simulink model "GisooLib"  (Simulink 8.1)
settings: Solver=ode45  StartTime=0.0  StopTime=10.0  RelTol=1e-3
libraries: commutil2 x54, xpclib x9, simulink x7, etargetslib x7, dspnetwork x7, GisooLib x1, commcrc2 x1
settings Model: Creator=behdad  LastModifiedBy=behdad
settings DataIOCC: SignalLoggingSaveFormat=Dataset
settings OptimizationCC: ExpressionDepthLimit=128
settings DebuggingCC: FcnCallInpInsideContextMsg=EnableAllAsError
settings GRTTargetCC: CombineOutputUpdateFcns=on  GRTInterface=off

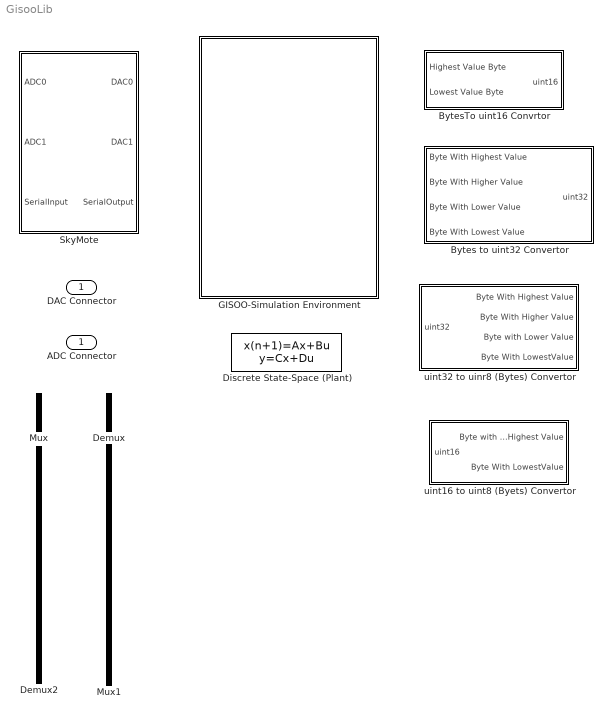
== system GisooLib ==
  ADC Connector : Inport
  Bytes to uint32 Convertor : Subsystem
  BytesTo uint16 Convrtor : Subsystem
  Demux : Demux  Outputs=2
  Demux2 : Demux  Outputs=16
  Discrete State-Space (Plant) : DiscreteStateSpace
  GISOO-Simulation Environment : Subsystem  TreatAsAtomicUnit=on
  Mux : Mux  Inputs=2
  Mux1 : Mux  Inputs=16
  SkyMote : Subsystem  mask{moteID=1, PacketType=6}
      mask prompts: PacketType "Serial Packet Type (Required block receives Serial data):"
  uint16 to uint8 (Byets) Convertor : Subsystem
  uint32 to uinr8 (Bytes) Convertor : Subsystem
  DAC Connector : Outport

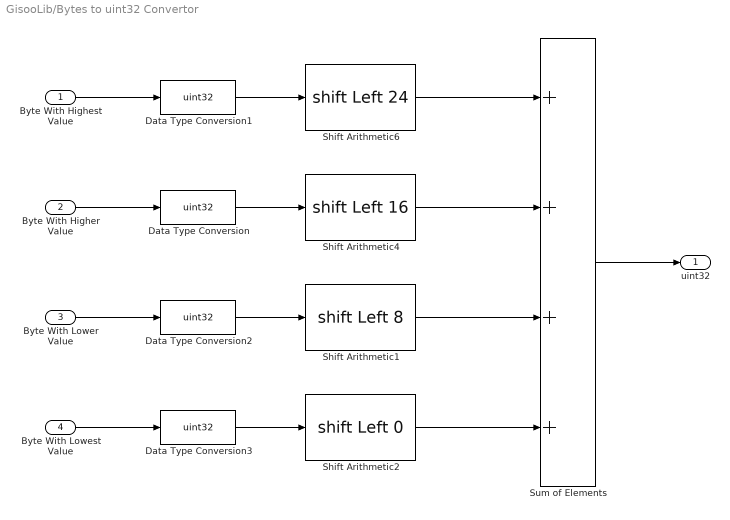
== system GisooLib/Bytes to uint32 Convertor ==
  Byte With Highest Value : Inport
  Byte With Higher Value : Inport  Port=2
  Byte With Lower Value : Inport  Port=3
  Byte With Lowest Value : Inport  Port=4
  Data Type Conversion{,1..3} (4 alike) : DataTypeConversion  OutDataTypeStr=uint32
  Shift Arithmetic1 : ArithShift  BitShiftNumber=8  BitShiftDirection=Left
  Shift Arithmetic2 : ArithShift  BitShiftDirection=Left
  Shift Arithmetic4 : ArithShift  BitShiftNumber=16  BitShiftDirection=Left
  Shift Arithmetic6 : ArithShift  BitShiftNumber=24  BitShiftDirection=Left
  Sum of Elements : Sum  Inputs=++++  CollapseDim=4  AccumDataTypeStr=uint8  OutDataTypeStr=uint32  InputSameDT=on
  uint32 : Outport
  wires:
  Data Type Conversion3/1 -> Shift Arithmetic2/1
  Shift Arithmetic1/1 -> Sum of Elements/3
  Shift Arithmetic6/1 -> Sum of Elements/1
  Byte With Lowest Value/1 -> Data Type Conversion3/1
  Shift Arithmetic2/1 -> Sum of Elements/4
  Byte With Lower Value/1 -> Data Type Conversion2/1
  Data Type Conversion2/1 -> Shift Arithmetic1/1
  Shift Arithmetic4/1 -> Sum of Elements/2
  Byte With Higher Value/1 -> Data Type Conversion/1
  Byte With Highest Value/1 -> Data Type Conversion1/1
  Data Type Conversion/1 -> Shift Arithmetic4/1
  Data Type Conversion1/1 -> Shift Arithmetic6/1
  Sum of Elements/1 -> uint32/1

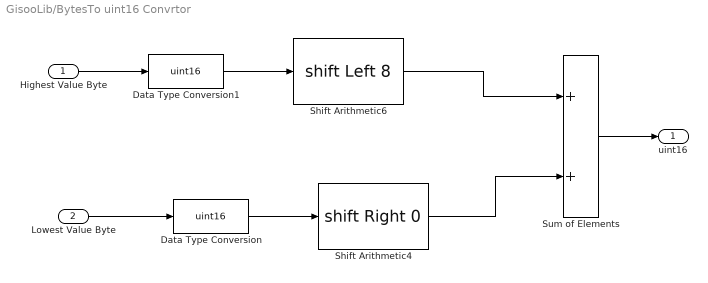
== system GisooLib/BytesTo uint16 Convrtor ==
  Highest Value Byte : Inport
  Lowest Value Byte : Inport  Port=2
  Data Type Conversion : DataTypeConversion  OutDataTypeStr=uint16
  Data Type Conversion1 : DataTypeConversion  OutDataTypeStr=uint16
  Shift Arithmetic4 : ArithShift  BitShiftDirection=Right
  Shift Arithmetic6 : ArithShift  BitShiftNumber=8  BitShiftDirection=Left
  Sum of Elements : Sum  CollapseDim=4  OutDataTypeStr=uint16
  uint16 : Outport
  wires:
  Lowest Value Byte/1 -> Data Type Conversion/1
  Highest Value Byte/1 -> Data Type Conversion1/1
  Data Type Conversion/1 -> Shift Arithmetic4/1
  Data Type Conversion1/1 -> Shift Arithmetic6/1
  Sum of Elements/1 -> uint16/1
  Shift Arithmetic4/1 -> Sum of Elements/2
  Shift Arithmetic6/1 -> Sum of Elements/1

== system GisooLib/GISOO-Simulation Environment ==
  CoojaConnector : Subsystem
  SynchronizerLoop : WhileIterator  MaxIters=-1  WhileBlockType=do-while  ShowIterationPort=on
  wires:
  CoojaConnector/1(Wait) -> SynchronizerLoop/1
  SynchronizerLoop/1 -> CoojaConnector/1(DelayNum.)

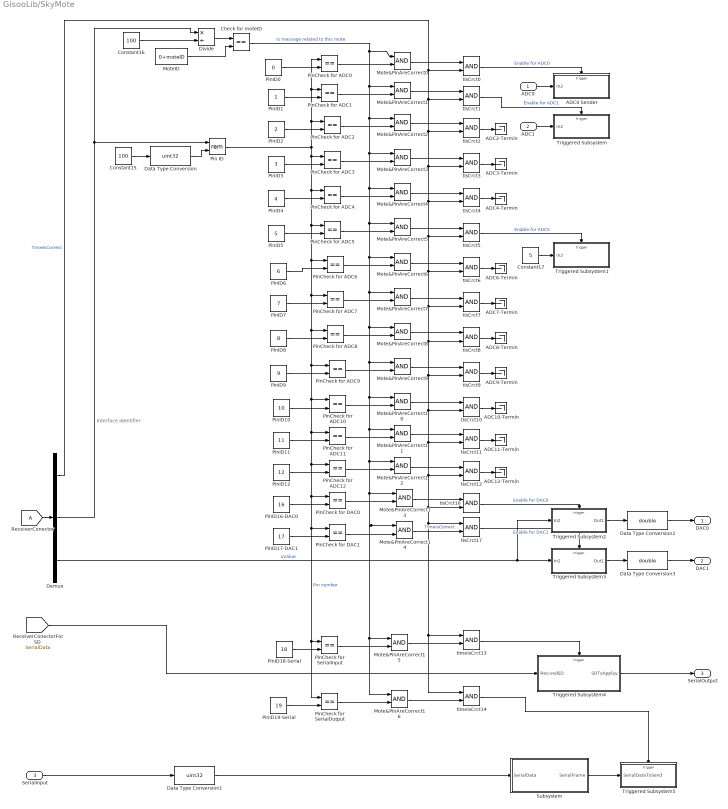
== system GisooLib/SkyMote ==
  note: Interface Identifier
  ADC0 : Inport
  ADC1 : Inport  Port=2
  SerialInput : Inport  Port=3
  ADC0 Sender : Subsystem  TreatAsAtomicUnit=on
  ADC10-Termin : Terminator
  ADC11-Termin : Terminator
  ADC12-Termin : Terminator
  ADC2-Termin : Terminator
  ADC3-Termin : Terminator
  ADC4-Termin : Terminator
  ADC6-Termin : Terminator
  ADC7-Termin : Terminator
  ADC8-Termin : Terminator
  ADC9-Termin : Terminator
  Check for moteID : RelationalOperator  Operator===  OutDataTypeStr=boolean
  Constant15 : Constant  Value=100
  Constant16 : Constant  Value=100
  Constant17 : Constant  Value=5
  Data Type Conversion : DataTypeConversion  OutDataTypeStr=uint32
  Data Type Conversion1 : DataTypeConversion  OutDataTypeStr=uint32
  Data Type Conversion2 : DataTypeConversion  OutDataTypeStr=double
  Data Type Conversion3 : DataTypeConversion  OutDataTypeStr=double
  Demux : Demux  Outputs=3
  Divide : Product  Inputs=*/  OutDataTypeStr=int32
  Mote&PinAreCorrect{0..16} (17 alike) : Logic  AllPortsSameDT=off  OutDataTypeStr=boolean
  MoteID : Constant  Value=0+moteID
  Pin ID : Math  Operator=rem  SaturateOnIntegerOverflow=on
  PinCheck for ADC{0..12} (13 alike) : RelationalOperator  Operator===  OutDataTypeStr=boolean
  PinCheck for DAC0 : RelationalOperator  Operator===  OutDataTypeStr=boolean
  PinCheck for DAC1 : RelationalOperator  Operator===  OutDataTypeStr=boolean
  PinCheck for SerialInput : RelationalOperator  Operator===  OutDataTypeStr=boolean
  PinCheck for SerialOutput : RelationalOperator  Operator===  OutDataTypeStr=boolean
  PinID0 : Constant  Value=0
  PinID1 : Constant
  PinID10 : Constant  Value=10
  PinID11 : Constant  Value=11
  PinID12 : Constant  Value=12
  PinID16-DAC0 : Constant  Value=16
  PinID17-DAC1 : Constant  Value=17
  PinID18-Serial : Constant  Value=18
  PinID19-Serial : Constant  Value=19
  PinID2 : Constant  Value=2
  PinID3 : Constant  Value=3
  PinID4 : Constant  Value=4
  PinID5 : Constant  Value=5
  PinID6 : Constant  Value=6
  PinID7 : Constant  Value=7
  PinID8 : Constant  Value=8
  PinID9 : Constant  Value=9
  Subsystem : Subsystem
  Triggered Subsystem : Subsystem  TreatAsAtomicUnit=on
  Triggered Subsystem1 : Subsystem  TreatAsAtomicUnit=on
  Triggered Subsystem2 : Subsystem  TreatAsAtomicUnit=on
  Triggered Subsystem3 : Subsystem  TreatAsAtomicUnit=on
  Triggered Subsystem4 : Subsystem  TreatAsAtomicUnit=on
  Triggered Subsystem5 : Subsystem  TreatAsAtomicUnit=on
  tIsCrct{0..12,16..17} (15 alike) : Logic  AllPortsSameDT=off  OutDataTypeStr=boolean
  timeIsCrct13 : Logic  AllPortsSameDT=off  OutDataTypeStr=boolean
  timeIsCrct14 : Logic  AllPortsSameDT=off  OutDataTypeStr=boolean
  DAC0 : Outport
  DAC1 : Outport  Port=2
  SerialOutput : Outport  Port=3
  wires:
  PinCheck for SerialInput/1 -> Mote&PinAreCorrect15/2
  Data Type Conversion1/1 -> Subsystem/1(SerialData)
  SerialInput/1 -> Data Type Conversion1/1
  timeIsCrct14/1 -> Triggered Subsystem5/Trigger
  Mote&PinAreCorrect16/1 -> timeIsCrct14/2
  PinCheck for SerialOutput/1 -> Mote&PinAreCorrect16/2
  PinID19-Serial/1 -> PinCheck for SerialOutput/2
  Check for moteID/1 -> Mote&PinAreCorrect0/1, Mote&PinAreCorrect2/1, Mote&PinAreCorrect3/1, Mote&PinAreCorrect4/1, Mote&PinAreCorrect5/1, Mote&PinAreCorrect6/1, Mote&PinAreCorrect7/1, Mote&PinAreCorrect8/1, Mote&PinAreCorrect9/1, Mote&PinAreCorrect10/1, Mote&PinAreCorrect11/1, Mote&PinAreCorrect12/1, Mote&PinAreCorrect15/1, Mote&PinAreCorrect16/1, Mote&PinAreCorrect14/1, Mote&PinAreCorrect13/1, Mote&PinAreCorrect1/1  "Is message related to this mote"
  Mote&PinAreCorrect15/1 -> timeIsCrct13/2
  Pin ID/1 -> PinCheck for ADC3/1, PinCheck for ADC4/1, PinCheck for ADC5/1, PinCheck for ADC6/1, PinCheck for ADC7/1, PinCheck for ADC8/1, PinCheck for ADC9/1, PinCheck for ADC10/1, PinCheck for ADC11/1, PinCheck for ADC12/1, PinCheck for DAC0/1, PinCheck for DAC1/1, PinCheck for SerialInput/1, PinCheck for SerialOutput/1, PinCheck for ADC2/1, PinCheck for ADC1/1, PinCheck for ADC0/1  "Pin number"
  tIsCrct12/1 -> ADC12-Termin/1
  Triggered Subsystem4/1(SDToApplay) -> SerialOutput/1
  Mote&PinAreCorrect14/1 -> tIsCrct17/2  "TimeIsCorrect"
  timeIsCrct13/1 -> Triggered Subsystem4/Trigger
  [SerialData] -> Triggered Subsystem4/1(RecivedSD)
  PinID18-Serial/1 -> PinCheck for SerialInput/2
  Demux/1 -> tIsCrct17/1, timeIsCrct13/1, timeIsCrct14/1, tIsCrct16/2, tIsCrct12/2, tIsCrct11/2, tIsCrct10/2, tIsCrct9/2, tIsCrct8/2, tIsCrct7/2, tIsCrct6/2, tIsCrct5/2, tIsCrct4/2, tIsCrct3/2, tIsCrct2/2, tIsCrct1/2, tIsCrct0/2  "TimeIsCorrect"
  Subsystem/1(SerialFrame) -> Triggered Subsystem5/1(SerialDataToSend)
  PinID17-DAC1/1 -> PinCheck for DAC1/2
  PinID16-DAC0/1 -> PinCheck for DAC0/2
  PinID12/1 -> PinCheck for ADC12/2
  PinID11/1 -> PinCheck for ADC11/2
  PinID9/1 -> PinCheck for ADC9/2
  PinID1/1 -> PinCheck for ADC1/2
  PinID10/1 -> PinCheck for ADC10/2
  PinID8/1 -> PinCheck for ADC8/2
  PinID7/1 -> PinCheck for ADC7/2
  PinID6/1 -> PinCheck for ADC6/2
  PinID5/1 -> PinCheck for ADC5/2
  PinID4/1 -> PinCheck for ADC4/2
  PinID3/1 -> PinCheck for ADC3/2
  PinID2/1 -> PinCheck for ADC2/2
  PinID0/1 -> PinCheck for ADC0/2
  PinCheck for ADC0/1 -> Mote&PinAreCorrect0/2
  PinCheck for ADC1/1 -> Mote&PinAreCorrect1/2
  PinCheck for ADC2/1 -> Mote&PinAreCorrect2/2
  PinCheck for ADC3/1 -> Mote&PinAreCorrect3/2
  PinCheck for ADC4/1 -> Mote&PinAreCorrect4/2
  PinCheck for ADC5/1 -> Mote&PinAreCorrect5/2
  PinCheck for ADC6/1 -> Mote&PinAreCorrect6/2
  PinCheck for ADC7/1 -> Mote&PinAreCorrect7/2
  PinCheck for ADC8/1 -> Mote&PinAreCorrect8/2
  PinCheck for ADC9/1 -> Mote&PinAreCorrect9/2
  PinCheck for ADC10/1 -> Mote&PinAreCorrect10/2
  PinCheck for ADC11/1 -> Mote&PinAreCorrect11/2
  PinCheck for ADC12/1 -> Mote&PinAreCorrect12/2
  PinCheck for DAC0/1 -> Mote&PinAreCorrect13/2
  PinCheck for DAC1/1 -> Mote&PinAreCorrect14/2
  Constant16/1 -> Divide/2
  Divide/1 -> Check for moteID/1
  MoteID/1 -> Check for moteID/2
  Mote&PinAreCorrect13/1 -> tIsCrct16/1
  Mote&PinAreCorrect12/1 -> tIsCrct12/1
  Mote&PinAreCorrect8/1 -> tIsCrct8/1
  Mote&PinAreCorrect7/1 -> tIsCrct7/1
  Mote&PinAreCorrect6/1 -> tIsCrct6/1
  Mote&PinAreCorrect4/1 -> tIsCrct4/1
  Mote&PinAreCorrect3/1 -> tIsCrct3/1
  Constant15/1 -> Data Type Conversion/1
  Data Type Conversion/1 -> Pin ID/2
  tIsCrct16/1 -> Triggered Subsystem2/Trigger  "Enable for DAC0"
  tIsCrct17/1 -> Triggered Subsystem3/Trigger  "Enable for DAC1"
  [A] -> Demux/1
  Demux/3 -> Triggered Subsystem3/1(In2), Triggered Subsystem2/1(In2)  "uValue"
  ADC0/1 -> ADC0 Sender/1(In2)
  Demux/2 -> Divide/1, Pin ID/1
  Data Type Conversion2/1 -> DAC0/1
  Triggered Subsystem2/1(Out1) -> Data Type Conversion2/1
  Data Type Conversion3/1 -> DAC1/1
  Triggered Subsystem3/1(Out1) -> Data Type Conversion3/1
  Constant17/1 -> Triggered Subsystem1/1(In2)
  Mote&PinAreCorrect0/1 -> tIsCrct0/1
  tIsCrct0/1 -> ADC0 Sender/Trigger  "Enable for ADC0"
  ADC1/1 -> Triggered Subsystem/1(In2)
  Mote&PinAreCorrect1/1 -> tIsCrct1/1
  tIsCrct1/1 -> Triggered Subsystem/Trigger  "Enable for ADC1"
  tIsCrct2/1 -> ADC2-Termin/1
  Mote&PinAreCorrect2/1 -> tIsCrct2/1
  tIsCrct3/1 -> ADC3-Termin/1
  tIsCrct4/1 -> ADC4-Termin/1
  tIsCrct6/1 -> ADC6-Termin/1
  Mote&PinAreCorrect5/1 -> tIsCrct5/1
  tIsCrct5/1 -> Triggered Subsystem1/Trigger  "Enable for ADC5"
  tIsCrct7/1 -> ADC7-Termin/1
  tIsCrct8/1 -> ADC8-Termin/1
  tIsCrct9/1 -> ADC9-Termin/1
  Mote&PinAreCorrect9/1 -> tIsCrct9/1
  tIsCrct10/1 -> ADC10-Termin/1
  Mote&PinAreCorrect10/1 -> tIsCrct10/1
  tIsCrct11/1 -> ADC11-Termin/1
  Mote&PinAreCorrect11/1 -> tIsCrct11/1

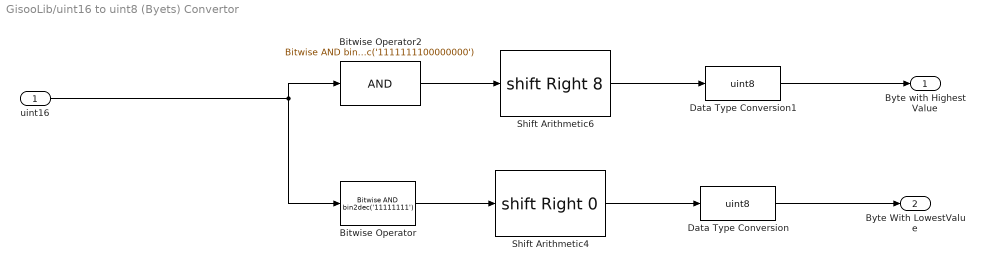
== system GisooLib/uint16 to uint8 (Byets) Convertor ==
  uint16 : Inport
  Bitwise Operator : simulink/Logic and Bit Operations/Bitwise Operator  logicop=AND  UseBitMask=on  BitMask=bin2dec('11111111')  BitMaskRealWorld=Stored Integer
  Bitwise Operator2 : simulink/Logic and Bit Operations/Bitwise Operator  logicop=AND  UseBitMask=on  BitMask=bin2dec('1111111100000000')  BitMaskRealWorld=Stored Integer
  Data Type Conversion : DataTypeConversion  OutDataTypeStr=uint8
  Data Type Conversion1 : DataTypeConversion  OutDataTypeStr=uint8
  Shift Arithmetic4 : ArithShift  BitShiftDirection=Right
  Shift Arithmetic6 : ArithShift  BitShiftNumber=8  BitShiftDirection=Right
  Byte with Highest Value : Outport
  Byte With LowestValue : Outport  Port=2
  wires:
  Bitwise Operator/1 -> Shift Arithmetic4/1
  Bitwise Operator2/1 -> Shift Arithmetic6/1
  Data Type Conversion1/1 -> Byte with Highest Value/1
  Shift Arithmetic4/1 -> Data Type Conversion/1
  Shift Arithmetic6/1 -> Data Type Conversion1/1
  uint16/1 -> Bitwise Operator/1, Bitwise Operator2/1
  Data Type Conversion/1 -> Byte With LowestValue/1

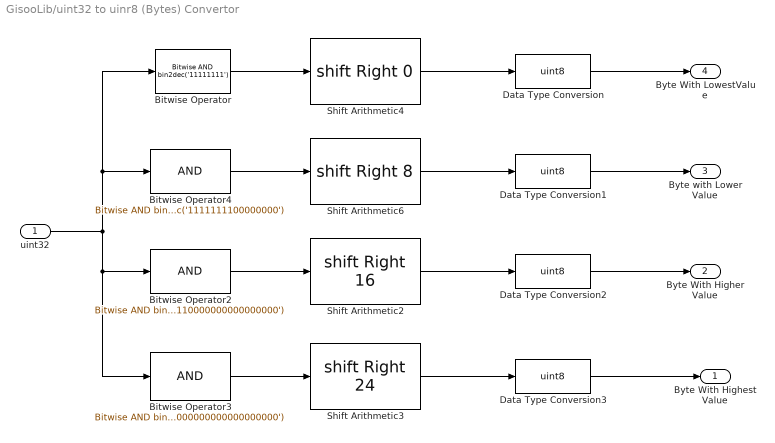
== system GisooLib/uint32 to uinr8 (Bytes) Convertor ==
  uint32 : Inport
  Bitwise Operator : simulink/Logic and Bit Operations/Bitwise Operator  logicop=AND  UseBitMask=on  BitMask=bin2dec('11111111')  BitMaskRealWorld=Stored Integer
  Bitwise Operator2 : simulink/Logic and Bit Operations/Bitwise Operator  logicop=AND  UseBitMask=on  BitMask=bin2dec('111111110000000000000000')  BitMaskRealWorld=Stored Integer
  Bitwise Operator3 : simulink/Logic and Bit Operations/Bitwise Operator  logicop=AND  UseBitMask=on  BitMask=bin2dec('11111111000000000000000000000000')  BitMaskRealWorld=Stored Integer
  Bitwise Operator4 : simulink/Logic and Bit Operations/Bitwise Operator  logicop=AND  UseBitMask=on  BitMask=bin2dec('1111111100000000')  BitMaskRealWorld=Stored Integer
  Data Type Conversion{,1..3} (4 alike) : DataTypeConversion  OutDataTypeStr=uint8
  Shift Arithmetic2 : ArithShift  BitShiftNumber=16  BitShiftDirection=Right
  Shift Arithmetic3 : ArithShift  BitShiftNumber=24  BitShiftDirection=Right
  Shift Arithmetic4 : ArithShift  BitShiftDirection=Right
  Shift Arithmetic6 : ArithShift  BitShiftNumber=8  BitShiftDirection=Right
  Byte With Highest Value : Outport
  Byte With Higher Value : Outport  Port=2
  Byte with Lower Value : Outport  Port=3
  Byte With LowestValue : Outport  Port=4
  wires:
  Bitwise Operator2/1 -> Shift Arithmetic2/1
  Data Type Conversion2/1 -> Byte With Higher Value/1
  Bitwise Operator/1 -> Shift Arithmetic4/1
  Data Type Conversion3/1 -> Byte With Highest Value/1
  Bitwise Operator3/1 -> Shift Arithmetic3/1
  Shift Arithmetic6/1 -> Data Type Conversion1/1
  Data Type Conversion1/1 -> Byte with Lower Value/1
  Data Type Conversion/1 -> Byte With LowestValue/1
  Shift Arithmetic2/1 -> Data Type Conversion2/1
  Shift Arithmetic4/1 -> Data Type Conversion/1
  uint32/1 -> Bitwise Operator4/1, Bitwise Operator/1, Bitwise Operator2/1, Bitwise Operator3/1
  Bitwise Operator4/1 -> Shift Arithmetic6/1
  Shift Arithmetic3/1 -> Data Type Conversion3/1

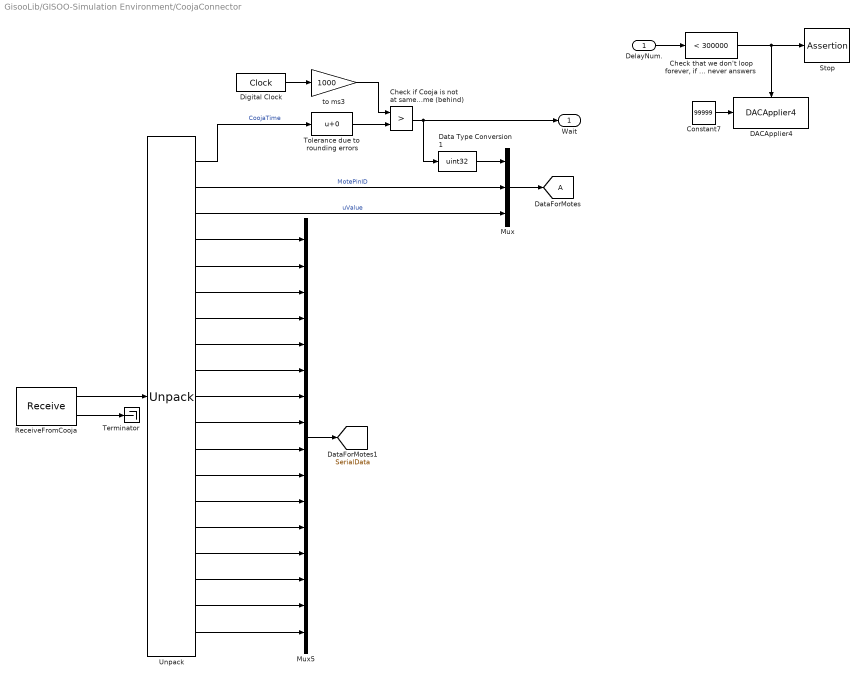
== system GisooLib/GISOO-Simulation Environment/CoojaConnector ==
  DelayNum. : Inport
  Check if Cooja is not at same time (behind) : RelationalOperator  Operator=>  OutDataTypeStr=boolean
  "Check that we don't loop forever, if Cooja never answers" : simulink/Logic and Bit Operations/Compare To Constant  relop=<  const=300000  OutDataTypeStr=uint8  ZeroCross=off
  Constant7 : Constant  Value=99999
  DACApplier4 : GisooLib/Cooja Platform/CoojaConnector/DACApplier4
  Data Type Conversion1 : DataTypeConversion  OutDataTypeStr=uint32
  Digital Clock : DigitalClock  SampleTime=-1
  Mux : Mux  Inputs=3
  Mux5 : Mux  Inputs=16
  ReceiveFromCooja : xpclib/UDP/Receive  ipAddress=127.0.0.1  ipPort=55555  width=28  vblLen=off  sampletime=-1
  Stop : Assertion  AssertionFailFcn=warning('No time-synchronization with ns-2');
  Terminator : Terminator
  Tolerance due to rounding errors : Bias
  Unpack : xpclib/UDP/Unpack  dimensions={[1],[1],[1],[1],[1],[1],[1],[1],[1],[1],[1],[1],[1],[1],[1],[1],[1],[1],[1]}  datatypes={'uint32','uint32','uint32','uint8','uint8','uint8','uint8','uint8','uint8','uint8','uint8','uint8','uint8','uint8','uint8','uint8','uint8','uint8','uint8'}  byteAlign=1
  to ms3 : Gain  Gain=1000  ParamDataTypeStr=uint32  OutDataTypeStr=Inherit: Inherit via back propagation
  Wait : Outport
  tag scope: A=global, SerialData=global
  wires:
  ReceiveFromCooja/1 -> Unpack/1
  to ms3/1 -> Check if Cooja is not at same time (behind)/1
  ReceiveFromCooja/2 -> Terminator/1
  Digital Clock/1 -> to ms3/1
  Unpack/10 -> Mux5/7
  Unpack/9 -> Mux5/6
  Unpack/8 -> Mux5/5
  Unpack/7 -> Mux5/4
  Unpack/6 -> Mux5/3
  Unpack/5 -> Mux5/2
  Unpack/4 -> Mux5/1
  Mux5/1 -> [SerialData]
  Constant7/1 -> DACApplier4/1
  Mux/1 -> [A]
  DelayNum./1 -> "Check that we don't loop forever, if Cooja never answers"/1
  "Check that we don't loop forever, if Cooja never answers"/1 -> Stop/1, DACApplier4/Trigger
  Data Type Conversion1/1 -> Mux/1
  Unpack/3 -> Mux/3  "uValue"
  Tolerance due to rounding errors/1 -> Check if Cooja is not at same time (behind)/2
  Unpack/1 -> Tolerance due to rounding errors/1  "CoojaTime"
  Unpack/2 -> Mux/2  "MotePinID"
  Check if Cooja is not at same time (behind)/1 -> Wait/1, Data Type Conversion1/1
  Unpack/11 -> Mux5/8
  Unpack/12 -> Mux5/9
  Unpack/13 -> Mux5/10
  Unpack/14 -> Mux5/11
  Unpack/15 -> Mux5/12
  Unpack/16 -> Mux5/13
  Unpack/17 -> Mux5/14
  Unpack/18 -> Mux5/15
  Unpack/19 -> Mux5/16

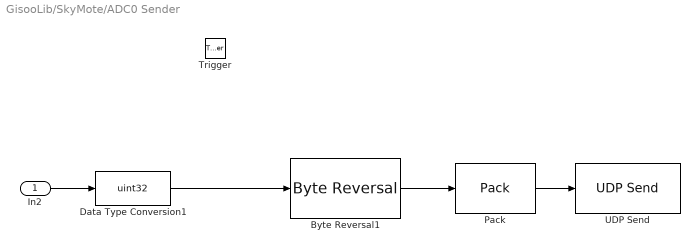
== system GisooLib/SkyMote/ADC0 Sender ==
  In2 : Inport
  Trigger : TriggerPort
  Byte Reversal1 : etargetslib/Byte Reversal  numInp=1
  Data Type Conversion1 : DataTypeConversion  OutDataTypeStr=uint32
  Pack : xpclib/UDP/Pack  datatypes={'uint32'}  byteAlign=1
  UDP Send : dspnetwork/UDP Send  remoteURL='127.0.0.1'  remotePort=18000+moteID  localURL='0.0.0.0'  localPortSource=Automatically determine  localPort=-1  sampletime=-1  separateLengthPort=0
  wires:
  Pack/1 -> UDP Send/1
  In2/1 -> Data Type Conversion1/1
  Byte Reversal1/1 -> Pack/1
  Data Type Conversion1/1 -> Byte Reversal1/1

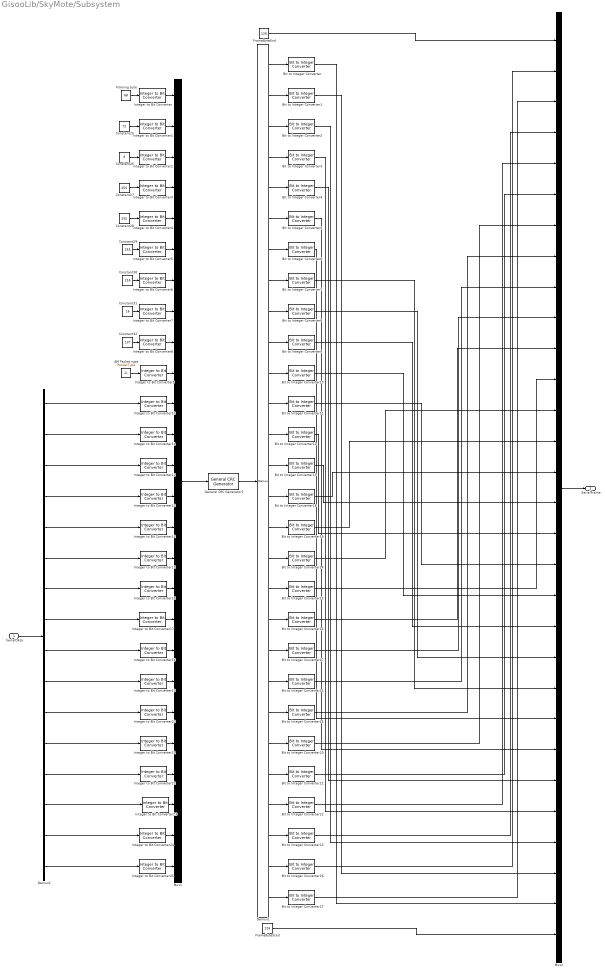
== system GisooLib/SkyMote/Subsystem ==
  SerialData : Inport
  AM Packet type : Constant  Value=PacketType  OutDataTypeStr=double
  Bit to Integer Converter{,1..27} (28 alike) : commutil2/Bit to Integer Converter  nbits=8  bitOrder=MSB first  signedOutputValues=Unsigned  outDtype=Inherit via internal rule  outDtypeSigned=Inherit via internal rule
  Constant25 : Constant  Value=72  OutDataTypeStr=double
  Constant26 : Constant  Value=0  OutDataTypeStr=double
  Constant{27..30} (4 alike) : Constant  Value=255  OutDataTypeStr=double
  Constant31 : Constant  Value=16  OutDataTypeStr=double
  Constant32 : Constant  Value=137  OutDataTypeStr=double
  Demux1 : Demux  Outputs=28
  Demux2 : Demux  Outputs=16
  FrameByteEnd : Constant  Value=126  OutDataTypeStr=uint8
  FrameByteStart : Constant  Value=126  OutDataTypeStr=uint8
  Framing byte : Constant  Value=68  OutDataTypeStr=uint8
  General CRC Generator1 : commcrc2/General CRC Generator  genPoly=[1 0 0 0 1 0 0 0 0 0 0 1 0 0 0 0 1]  iniStates=0  directMethod=off  reflectInputBytes=off  reflectChecksums=off  finalXOR=0  numChecksums=1
  Integer to Bit Converter{,1..25} (26 alike) : commutil2/Integer to Bit Converter  nbits=8  signedInputValues=Unsigned  bitOrder=MSB first  outDtype=boolean
  Mux1 : Mux  Inputs=26
  Mux2 : Mux  Inputs=30
  SerialFrame : Outport
  wires:
  Bit to Integer Converter23/1 -> Mux2/4
  Bit to Integer Converter3/1 -> Mux2/26
  Demux2/4 -> Integer to Bit Converter13/1
  Bit to Integer Converter24/1 -> Mux2/9
  Bit to Integer Converter8/1 -> Mux2/21
  Demux2/3 -> Integer to Bit Converter12/1
  Bit to Integer Converter18/1 -> Mux2/15
  Bit to Integer Converter12/1 -> Mux2/17
  Bit to Integer Converter19/1 -> Mux2/14
  Bit to Integer Converter14/1 -> Mux2/13
  Demux2/7 -> Integer to Bit Converter16/1
  Bit to Integer Converter5/1 -> Mux2/24
  Bit to Integer Converter2/1 -> Mux2/27
  Bit to Integer Converter16/1 -> Mux2/11
  Bit to Integer Converter13/1 -> Mux2/16
  Bit to Integer Converter15/1 -> Mux2/12
  Bit to Integer Converter25/1 -> Mux2/8
  Bit to Integer Converter10/1 -> Mux2/19
  Bit to Integer Converter6/1 -> Mux2/23
  Bit to Integer Converter1/1 -> Mux2/28
  Bit to Integer Converter4/1 -> Mux2/25
  Bit to Integer Converter11/1 -> Mux2/18
  Bit to Integer Converter7/1 -> Mux2/22
  Bit to Integer Converter9/1 -> Mux2/20
  Bit to Integer Converter/1 -> Mux2/29
  Bit to Integer Converter20/1 -> Mux2/7
  Bit to Integer Converter17/1 -> Mux2/10
  Demux2/1 -> Integer to Bit Converter10/1
  Demux2/2 -> Integer to Bit Converter11/1
  Bit to Integer Converter21/1 -> Mux2/6
  SerialData/1 -> Demux2/1
  Bit to Integer Converter22/1 -> Mux2/5
  Demux2/5 -> Integer to Bit Converter14/1
  Demux2/6 -> Integer to Bit Converter15/1
  Integer to Bit Converter14/1 -> Mux1/15
  Integer to Bit Converter24/1 -> Mux1/25
  Integer to Bit Converter23/1 -> Mux1/24
  Integer to Bit Converter11/1 -> Mux1/12
  Constant30/1 -> Integer to Bit Converter6/1
  Demux1/10 -> Bit to Integer Converter9/1
  Demux1/8 -> Bit to Integer Converter7/1
  Integer to Bit Converter13/1 -> Mux1/14
  Integer to Bit Converter17/1 -> Mux1/18
  Integer to Bit Converter15/1 -> Mux1/16
  Integer to Bit Converter16/1 -> Mux1/17
  Demux1/2 -> Bit to Integer Converter1/1
  Integer to Bit Converter6/1 -> Mux1/7
  Demux2/10 -> Integer to Bit Converter19/1
  Integer to Bit Converter10/1 -> Mux1/11
  Demux2/8 -> Integer to Bit Converter17/1
  Constant25/1 -> Integer to Bit Converter1/1
  Demux2/12 -> Integer to Bit Converter21/1
  Integer to Bit Converter/1 -> Mux1/1
  Demux2/13 -> Integer to Bit Converter22/1
  Demux2/15 -> Integer to Bit Converter24/1
  Framing byte/1 -> Integer to Bit Converter/1
  Mux1/1 -> General CRC Generator1/1
  Demux2/16 -> Integer to Bit Converter25/1
  Demux2/14 -> Integer to Bit Converter23/1
  Integer to Bit Converter5/1 -> Mux1/6
  Integer to Bit Converter1/1 -> Mux1/2
  Constant29/1 -> Integer to Bit Converter5/1
  Constant26/1 -> Integer to Bit Converter2/1
  Constant27/1 -> Integer to Bit Converter3/1
  Integer to Bit Converter4/1 -> Mux1/5
  Constant28/1 -> Integer to Bit Converter4/1
  Integer to Bit Converter3/1 -> Mux1/4
  Integer to Bit Converter2/1 -> Mux1/3
  Demux1/3 -> Bit to Integer Converter2/1
  Integer to Bit Converter7/1 -> Mux1/8
  General CRC Generator1/1 -> Demux1/1
  Integer to Bit Converter8/1 -> Mux1/9
  Constant32/1 -> Integer to Bit Converter8/1
  Integer to Bit Converter25/1 -> Mux1/26
  Integer to Bit Converter21/1 -> Mux1/22
  Integer to Bit Converter22/1 -> Mux1/23
  FrameByteEnd/1 -> Mux2/1
  AM Packet type/1 -> Integer to Bit Converter9/1
  Demux1/11 -> Bit to Integer Converter10/1
  Demux2/11 -> Integer to Bit Converter20/1
  Demux1/1 -> Bit to Integer Converter/1
  Demux1/9 -> Bit to Integer Converter8/1
  Demux1/13 -> Bit to Integer Converter12/1
  Demux1/7 -> Bit to Integer Converter6/1
  Demux2/9 -> Integer to Bit Converter18/1
  Integer to Bit Converter12/1 -> Mux1/13
  Mux2/1 -> SerialFrame/1
  Demux1/12 -> Bit to Integer Converter11/1
  Integer to Bit Converter18/1 -> Mux1/19
  Integer to Bit Converter9/1 -> Mux1/10
  Integer to Bit Converter20/1 -> Mux1/21
  Integer to Bit Converter19/1 -> Mux1/20
  Constant31/1 -> Integer to Bit Converter7/1
  Demux1/24 -> Bit to Integer Converter21/1
  Demux1/4 -> Bit to Integer Converter3/1
  Demux1/21 -> Bit to Integer Converter24/1
  Demux1/5 -> Bit to Integer Converter4/1
  Demux1/19 -> Bit to Integer Converter16/1
  Demux1/20 -> Bit to Integer Converter17/1
  Demux1/23 -> Bit to Integer Converter20/1
  Demux1/22 -> Bit to Integer Converter25/1
  Demux1/26 -> Bit to Integer Converter23/1
  Demux1/18 -> Bit to Integer Converter15/1
  Demux1/17 -> Bit to Integer Converter14/1
  Demux1/25 -> Bit to Integer Converter22/1
  Demux1/16 -> Bit to Integer Converter19/1
  Demux1/6 -> Bit to Integer Converter5/1
  Demux1/14 -> Bit to Integer Converter13/1
  Demux1/15 -> Bit to Integer Converter18/1
  Demux1/27 -> Bit to Integer Converter26/1
  Bit to Integer Converter26/1 -> Mux2/2
  FrameByteStart/1 -> Mux2/30
  Demux1/28 -> Bit to Integer Converter27/1
  Bit to Integer Converter27/1 -> Mux2/3

== system GisooLib/SkyMote/Triggered Subsystem ==
  In2 : Inport
  Trigger : TriggerPort
  Byte Reversal1 : etargetslib/Byte Reversal  numInp=1
  Data Type Conversion1 : DataTypeConversion  OutDataTypeStr=uint32
  Pack : xpclib/UDP/Pack  datatypes={'uint32'}  byteAlign=1
  UDP Send : dspnetwork/UDP Send  remoteURL='127.0.0.1'  remotePort=18000+moteID  localURL='0.0.0.0'  localPortSource=Automatically determine  localPort=-1  sampletime=-1  separateLengthPort=0
  wires:
  In2/1 -> Data Type Conversion1/1
  Pack/1 -> UDP Send/1
  Byte Reversal1/1 -> Pack/1
  Data Type Conversion1/1 -> Byte Reversal1/1

== system GisooLib/SkyMote/Triggered Subsystem1 ==
  In2 : Inport
  Trigger : TriggerPort
  Byte Reversal1 : etargetslib/Byte Reversal  numInp=1
  Data Type Conversion1 : DataTypeConversion  OutDataTypeStr=uint32
  Pack : xpclib/UDP/Pack  datatypes={'uint32'}  byteAlign=1
  UDP Send : dspnetwork/UDP Send  remoteURL='127.0.0.1'  remotePort=18000+moteID  localURL='0.0.0.0'  localPortSource=Automatically determine  localPort=-1  sampletime=-1  separateLengthPort=0
  wires:
  Pack/1 -> UDP Send/1
  In2/1 -> Data Type Conversion1/1
  Data Type Conversion1/1 -> Byte Reversal1/1
  Byte Reversal1/1 -> Pack/1

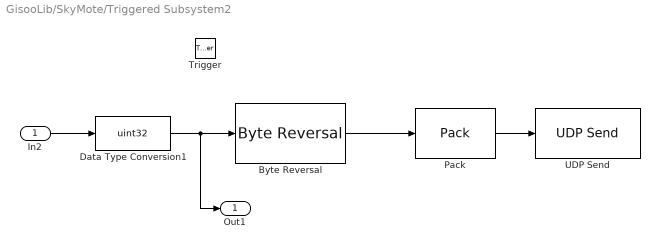
== system GisooLib/SkyMote/Triggered Subsystem2 ==
  In2 : Inport
  Trigger : TriggerPort
  Byte Reversal : etargetslib/Byte Reversal  numInp=1
  Data Type Conversion1 : DataTypeConversion  OutDataTypeStr=uint32
  Pack : xpclib/UDP/Pack  datatypes={'uint32'}  byteAlign=1
  UDP Send : dspnetwork/UDP Send  remoteURL='127.0.0.1'  remotePort=18000+moteID  localURL='0.0.0.0'  localPortSource=Automatically determine  localPort=-1  sampletime=-1  separateLengthPort=0
  Out1 : Outport
  wires:
  In2/1 -> Data Type Conversion1/1
  Data Type Conversion1/1 -> Out1/1, Byte Reversal/1
  Pack/1 -> UDP Send/1
  Byte Reversal/1 -> Pack/1

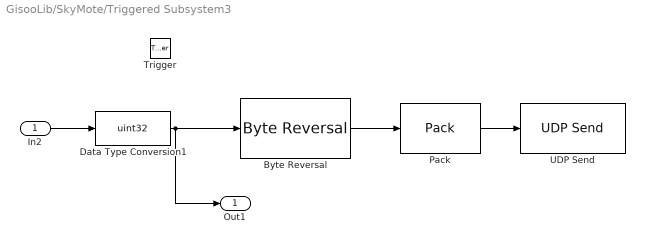
== system GisooLib/SkyMote/Triggered Subsystem3 ==
  In2 : Inport
  Trigger : TriggerPort
  Byte Reversal : etargetslib/Byte Reversal  numInp=1
  Data Type Conversion1 : DataTypeConversion  OutDataTypeStr=uint32
  Pack : xpclib/UDP/Pack  datatypes={'uint32'}  byteAlign=1
  UDP Send : dspnetwork/UDP Send  remoteURL='127.0.0.1'  remotePort=18000+moteID  localURL='0.0.0.0'  localPortSource=Automatically determine  localPort=-1  sampletime=-1  separateLengthPort=0
  Out1 : Outport
  wires:
  Pack/1 -> UDP Send/1
  Data Type Conversion1/1 -> Byte Reversal/1, Out1/1
  In2/1 -> Data Type Conversion1/1
  Byte Reversal/1 -> Pack/1

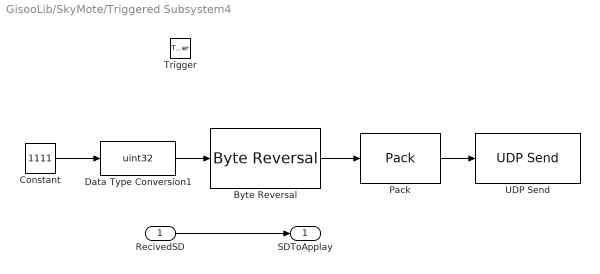
== system GisooLib/SkyMote/Triggered Subsystem4 ==
  RecivedSD : Inport
  Trigger : TriggerPort
  Byte Reversal : etargetslib/Byte Reversal  numInp=1
  Constant : Constant  Value=1111
  Data Type Conversion1 : DataTypeConversion  OutDataTypeStr=uint32
  Pack : xpclib/UDP/Pack  datatypes={'uint32'}  byteAlign=1
  UDP Send : dspnetwork/UDP Send  remoteURL='127.0.0.1'  remotePort=18000+moteID  localURL='0.0.0.0'  localPortSource=Automatically determine  localPort=-1  sampletime=-1  separateLengthPort=0
  SDToApplay : Outport
  wires:
  Pack/1 -> UDP Send/1
  RecivedSD/1 -> SDToApplay/1
  Constant/1 -> Data Type Conversion1/1
  Byte Reversal/1 -> Pack/1
  Data Type Conversion1/1 -> Byte Reversal/1

== system GisooLib/SkyMote/Triggered Subsystem5 ==
  SerialDataToSend : Inport
  Trigger : TriggerPort
  Byte Reversal : etargetslib/Byte Reversal  numInp=1
  Demux : Demux  Outputs=30
  Pack : xpclib/UDP/Pack  datatypes={'uint8','uint8','uint8','uint8','uint8','uint8','uint8','uint8','uint8','uint8','uint8','uint8','uint8','uint8','uint8','uint8','uint8','uint8','uint8','uint8','uint8','uint8','uint8','uint8','uint8','uint8','uint8','uint8','uint8','uint8'}  byteAlign=1
  UDP Send : dspnetwork/UDP Send  remoteURL='127.0.0.1'  remotePort=18000+moteID  localURL='0.0.0.0'  localPortSource=Automatically determine  localPort=-1  sampletime=-1  separateLengthPort=0
  wires:
  Byte Reversal/1 -> Demux/1
  SerialDataToSend/1 -> Byte Reversal/1
  Demux/30 -> Pack/30
  Demux/29 -> Pack/29
  Demux/28 -> Pack/28
  Demux/27 -> Pack/27
  Demux/26 -> Pack/26
  Demux/25 -> Pack/25
  Demux/24 -> Pack/24
  Demux/23 -> Pack/23
  Demux/22 -> Pack/22
  Demux/21 -> Pack/21
  Demux/20 -> Pack/20
  Demux/19 -> Pack/19
  Demux/18 -> Pack/18
  Demux/17 -> Pack/17
  Demux/16 -> Pack/16
  Demux/15 -> Pack/15
  Demux/14 -> Pack/14
  Demux/13 -> Pack/13
  Demux/12 -> Pack/12
  Demux/11 -> Pack/11
  Demux/10 -> Pack/10
  Demux/9 -> Pack/9
  Demux/8 -> Pack/8
  Demux/7 -> Pack/7
  Demux/6 -> Pack/6
  Demux/5 -> Pack/5
  Demux/4 -> Pack/4
  Demux/3 -> Pack/3
  Demux/2 -> Pack/2
  Demux/1 -> Pack/1
  Pack/1 -> UDP Send/1
